simulink model "X_SimulinkModell_GUI"  (R2018b)
settings: Solver=VariableStepAuto  StartTime=0.0  StopTime=0.2  FixedStep=0.0001  RelTol=1e-3  EnableMultiTasking=on
values from neighbouring files (symbols this model uses):
  F_Normal = (m_MagPol+m_Lauferstange)*9.81    [Simulink_Rand.m]
  final_para = [-8 12 18 40 10 1 5.5 39.5 20 4 7.5 1.195 ... (5610 elements, 30x187)]    [simulink_kennfelder_altermagnet.mat]    (also in simulink_kennfelder_altermagnet_ges.mat; simulink_kennfelder_neuermagnet.mat)
  I_max = [-20 -16 -12 -8 -4 0 4 8 12 16 20]    [simulink_kennfelder_altermagnet_ges.mat]
  Kraftbedarf =     [Kraftbedarf.mat]
  Kraftbedarf_gespiegelt =     [Kraftbedarf_gespiegelt.mat]
  KraftWegStrom = KraftWegStrom'    [Simulink_Rand.m]    (also in simulink_kennfelder_altermagnet.mat = [-12.365 -12.724 -13.215 -13.344 -14.014 -14.494 -14.248 -14; simulink_kennfelder_altermagnet_ges.mat = [-12.365 -12.724 -13.215 -13.344 -14.014 -14.494 -14.248 -14; simulink_kennfelder_neuermagnet.mat = [-13.233 -13.572 -14.313 -14.247 -14.812 -15.568 -15.262 -15)
  m_Ges = m_MagPol+m_Lauferstange+m_Kupplung+m_Schaltgabel_Muffe    [Simulink_Rand.m]
  mu_haft = 1.66    [Simulink_Rand.m]
  mu_reib = 1.19    [Simulink_Rand.m]
  pos = [-8 -7 -6 -5 -4 -3 -2 -1 0 1 2 3 ... (17 elements, 1x17)]    [simulink_kennfelder_altermagnet_ges.mat]
  R_Spule = (final_para(2)+2*final_para(3)+2*final_para(6)+final_para(7))*2*pi*final_para(13)*10^(-3)*final_para(18)    [Simulink_Rand.m]
undefined symbols (not defined in the file or in its folder): Flux
libraries: simulink x4
settings Model: Creator=adp_schaltaktorik  LastModifiedBy=ohahn
settings SolverCC: ZeroCrossAlgorithm=Adaptive
settings DataIOCC: LimitDataPoints=on  SaveFormat=Array  SaveTime=off
settings OptimizationCC: LifeSpan=inf
settings DebuggingCC: IgnoredZcDiagnostic=none  SolverPrmCheckMsg=warning  MultiTaskDSMMsg=warning  MultiTaskCondExecSysMsg=none  SFUnexpectedBacktrackingDiag=warning  SFNoUnconditionalDefaultTransitionDiag=warning  SFExecutionAtInitializationDiag=none
settings HardwareCC: ProdBitPerPointer=32  ProdBitPerSizeT=32  ProdBitPerPtrDiffT=32  ProdLargestAtomicFloat=None  ProdIntDivRoundTo=Undefined  ProdEndianess=Unspecified  ProdWordSize=32  ProdHWDeviceType=32-bit Generic
settings ModelReferenceCC: PropagateSignalLabelsOutOfModel=off
settings SFSimCC: SimUseLocalCustomCode=off
settings RTWCC: RTWUseLocalCustomCode=off
settings CodeAppCC: StateflowObjectComments=on
settings GRTTargetCC: TargetLangStandard=C89/C90 (ANSI)  GeneratePreprocessorConditionals=Disable all
settings ConfigComp: CovMetricSettings=dw  CovHtmlReporting=on  CovSaveCumulativeToWorkspaceVar=on  CovSaveSingleToWorkspaceVar=on  CovExternalEMLEnable=off
settings SimscapeCC: SimscapeNormalizeSystem=off

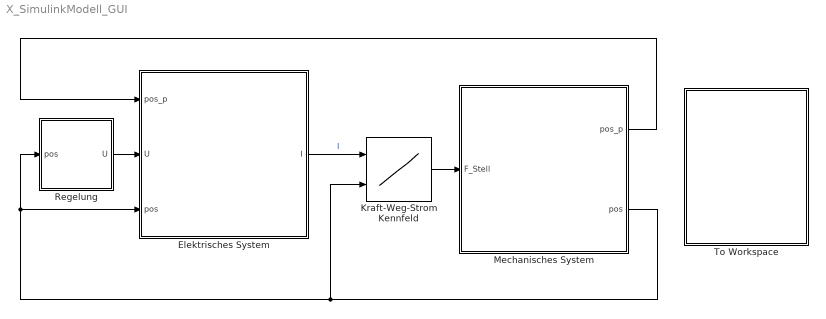
== system X_SimulinkModell_GUI ==
  Elektrisches System : Subsystem
  Kraft-Weg-Strom Kennfeld : Lookup_n-D  BreakpointsForDimension1=I_max  BreakpointsForDimension2=pos  Table=KraftWegStrom*10  InternalRulePriority=Speed  RndMeth=Simplest  InputSameDT=on
  Mechanisches System : Subsystem
  Regelung : Subsystem
  To Workspace : Subsystem
  wires:
  Mechanisches System/2(pos) -> Regelung/1("pos "), Elektrisches System/3(pos), Kraft-Weg-Strom Kennfeld/2
  Regelung/1(U) -> Elektrisches System/2(U)
  Elektrisches System/1(I) -> Kraft-Weg-Strom Kennfeld/1  "I"
  Kraft-Weg-Strom Kennfeld/1 -> Mechanisches System/1("F_Stell ")
  Mechanisches System/1("pos_p ") -> Elektrisches System/1(pos_p)

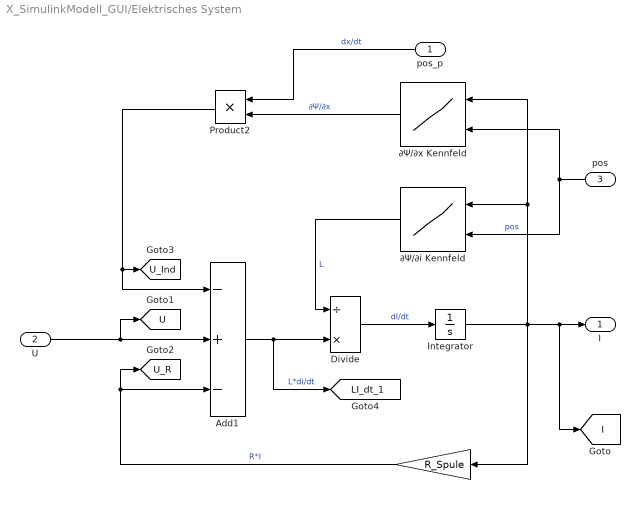
== system X_SimulinkModell_GUI/Elektrisches System ==
  pos_p : Inport
  U : Inport  Port=2
  pos : Inport  Port=3
  " " : Gain  Gain=R_Spule
  Add1 : Sum  Inputs=-+-
  Divide : Product  Inputs=/*
  Integrator : Integrator
  Product2 : Product
  "∂Ψ/∂i Kennfeld " : Lookup_n-D  BreakpointsForDimension1=Flux.i_zwischen  BreakpointsForDimension2=Flux.x  Table=Flux.phi_p_i*10  InternalRulePriority=Speed  RndMeth=Simplest  InputSameDT=on
  ∂Ψ/∂x Kennfeld : Lookup_n-D  BreakpointsForDimension1=Flux.i  BreakpointsForDimension2=Flux.x_zwischen  Table=Flux.phi_p_x*10  InternalRulePriority=Speed  RndMeth=Simplest  InputSameDT=on
  I : Outport
  tag scope: I=global, LI_dt_1=global, U=global, U_Ind=global, U_R=global
  wires:
  " "/1 -> Add1/3, [U_R]  "R*I"
  Add1/1 -> Divide/2, [LI_dt_1]  "L*di/dt"
  Divide/1 -> Integrator/1  "dI/dt"
  U/1 -> [U], Add1/2
  ∂Ψ/∂x Kennfeld/1 -> Product2/2  "∂Ψ/∂x"
  pos_p/1 -> Product2/1  "dx/dt"
  pos/1 -> "∂Ψ/∂i Kennfeld "/2, ∂Ψ/∂x Kennfeld/2  "pos"
  Product2/1 -> Add1/1, [U_Ind]
  Integrator/1 -> "∂Ψ/∂i Kennfeld "/1, ∂Ψ/∂x Kennfeld/1, [I], I/1, " "/1
  "∂Ψ/∂i Kennfeld "/1 -> Divide/1  "L"

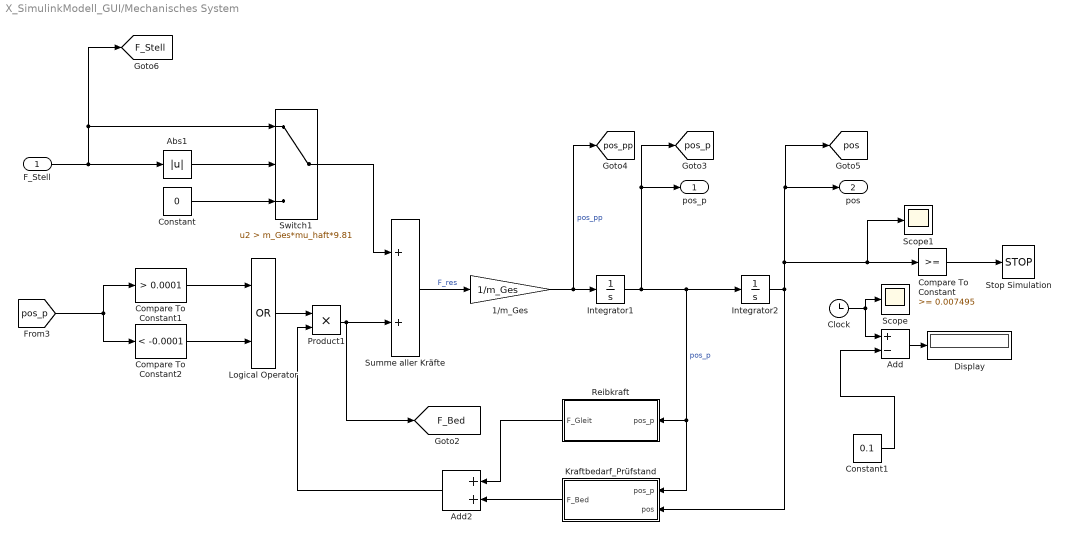
== system X_SimulinkModell_GUI/Mechanisches System ==
  "F_Stell " : Inport
  1/m_Ges : Gain  Gain=1/m_Ges
  Abs1 : Abs
  Add : Sum  Inputs=+-
  Add2 : Sum
  Clock : Clock
  Compare To Constant : simulink/Logic and Bit Operations/Compare To Constant  relop=>=  const=0.007495  OutDataTypeStr=boolean
  Compare To Constant1 : simulink/Logic and Bit Operations/Compare To Constant  relop=>  const=0.0001  OutDataTypeStr=boolean
  Compare To Constant2 : simulink/Logic and Bit Operations/Compare To Constant  relop=<  const=-0.0001  OutDataTypeStr=boolean
  Constant : Constant  Value=0
  Constant1 : Constant  Value=0.1
  Display : Display
  Integrator1 : Integrator
  Integrator2 : Integrator
  Kraftbedarf_Prüfstand : Subsystem
  Logical Operator : Logic  Operator=OR  AllPortsSameDT=off  OutDataTypeStr=boolean
  Product1 : Product
  Reibkraft : Subsystem
  Scope : Scope
  Scope1 : Scope
  Stop Simulation : Stop
  Summe aller Kräfte : Sum
  Switch1 : Switch  Criteria=u2 > Threshold  Threshold=m_Ges*mu_haft*9.81
  "pos_p " : Outport
  pos : Outport  Port=2
  tag scope: F_Bed=global, F_Stell=global, pos=global, pos_p=global, pos_pp=global
  wires:
  Integrator1/1 -> Integrator2/1, Reibkraft/1(pos_p), Kraftbedarf_Prüfstand/1(pos_p), "pos_p "/1, [pos_p]  "pos_p"
  1/m_Ges/1 -> [pos_pp], Integrator1/1  "pos_pp"
  Summe aller Kräfte/1 -> 1/m_Ges/1  "F_res"
  "F_Stell "/1 -> [F_Stell], Switch1/1, Abs1/1
  Integrator2/1 -> pos/1, [pos], Scope1/1, Compare To Constant/1, Kraftbedarf_Prüfstand/2(pos)
  Add2/1 -> Product1/2
  Abs1/1 -> Switch1/2
  Constant/1 -> Switch1/3
  Switch1/1 -> Summe aller Kräfte/1
  [pos_p] -> Compare To Constant1/1, Compare To Constant2/1
  Compare To Constant1/1 -> Logical Operator/1
  Logical Operator/1 -> Product1/1
  Reibkraft/1(F_Gleit) -> Add2/1
  Kraftbedarf_Prüfstand/1(F_Bed) -> Add2/2
  Compare To Constant2/1 -> Logical Operator/2
  Product1/1 -> [F_Bed], Summe aller Kräfte/2
  Compare To Constant/1 -> Stop Simulation/1
  Add/1 -> Display/1
  Constant1/1 -> Add/2
  Clock/1 -> Scope/1, Add/1

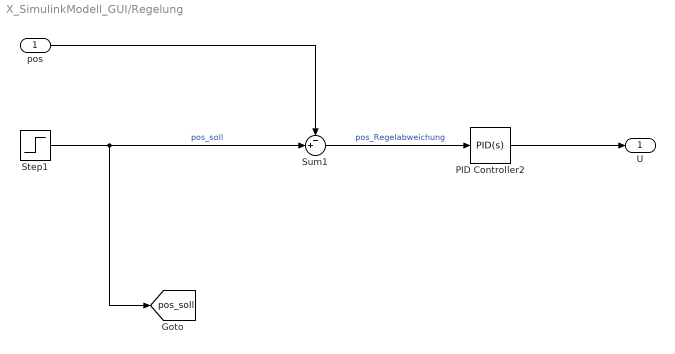
== system X_SimulinkModell_GUI/Regelung ==
  "pos " : Inport
  PID Controller2 : simulink/Continuous/PID Controller  Controller=PID  Form=Parallel  TimeDomain=Continuous-time  SampleTime=-1  IntegratorMethod=Forward Euler  FilterMethod=Forward Euler  ControllerParametersSource=internal  P=1480  I=9200  D=0  UseFilter=on  N=0  TunerSelectOption=Transfer Function Based (PID Tuner App)  InitialConditionSource=internal  InitialConditionForIntegrator=0  InitialConditionForFilter=0  DifferentiatorICPrevScaledInput=0  ExternalReset=none  TrackingMode=off  Kt=1  LimitOutput=on  UpperSaturationLimit=12  LowerSaturationLimit=-12  LinearizeAsGain=on  AntiWindupMode=none  Kb=1  POutMin=[]  POutMax=[]  IOutMin=[]  IOutMax=[]  DOutMin=[]  DOutMax=[]  NOutMin=[]  NOutMax=[]  SumOutMin=[]  SumOutMax=[]  SaturationOutMin=[]  SaturationOutMax=[]  PParamMin=[]  PParamMax=[]  IParamMin=[]  IParamMax=[]  DParamMin=[]  DParamMax=[]  NParamMin=[]  NParamMax=[]  KbParamMin=[]  KbParamMax=[]  KtParamMin=[]  KtParamMax=[]  KbOutMin=[]  KbOutMax=[]  KtOutMin=[]  KtOutMax=[]  IntegratorOutMin=[]  IntegratorOutMax=[]  FilterOutMin=[]  FilterOutMax=[]  SumI1OutMin=[]  SumI1OutMax=[]  SumI2OutMin=[]  SumI2OutMax=[]  SumI3OutMin=[]  SumI3OutMax=[]  SumI4OutMin=[]  SumI4OutMax=[]  SumDOutMin=[]  SumDOutMax=[]  DifferentiatorOutMin=[]  DifferentiatorOutMax=[]  FilterDiffOutCoefMin=[]  FilterDiffOutCoefMax=[]  ReciprocalOutMin=[]  ReciprocalOutMax=[]  SumDenOutMin=[]  SumDenOutMax=[]  SumNumOutMin=[]  SumNumOutMax=[]  DivideOutMin=[]  DivideOutMax=[]  IntegratorContinuousStateAttributes=''  IntegratorStateMustResolveToSignalObject=off  IntegratorRTWStateStorageClass=Auto  FilterContinuousStateAttributes=''  FilterStateMustResolveToSignalObject=off  FilterRTWStateStorageClass=Auto  ParallelPVariant=InternalParameters  IdealPVariant=Disabled  IVariant=InternalParameters  DVariant=InternalParameters  IntegratorVariant=Continuous  SatVariant=Enabled  AWVariant=Passthrough  PCopyVariant=Disabled  TRVariant=Disabled  FdbkBlocksVariant=Forward  IdealPFdbkVariant=Disabled  SatFdbkVariant=Disabled  DerivativeFilterVariant=ContFilter  NVariant=InternalParameters  NCopyVariant=Disabled  FilterICVariant=InternalICsFilter  IntegratorICVariant=InternalICs  ExternalResetVariant=Disabled  TRSumVariant=Passthrough  SumFdbkVariant=Disabled  SumVariant=Sum_PID
  Step1 : Step  Time=0.1  After=final_para(19)/2*0.001  SampleTime=0
  Sum1 : Sum  Inputs=-+|
  U : Outport
  tag scope: pos_soll=global
  wires:
  Step1/1 -> Sum1/2, [pos_soll]  "pos_soll"
  Sum1/1 -> PID Controller2/1  "pos_Regelabweichung"
  "pos "/1 -> Sum1/1
  PID Controller2/1 -> U/1

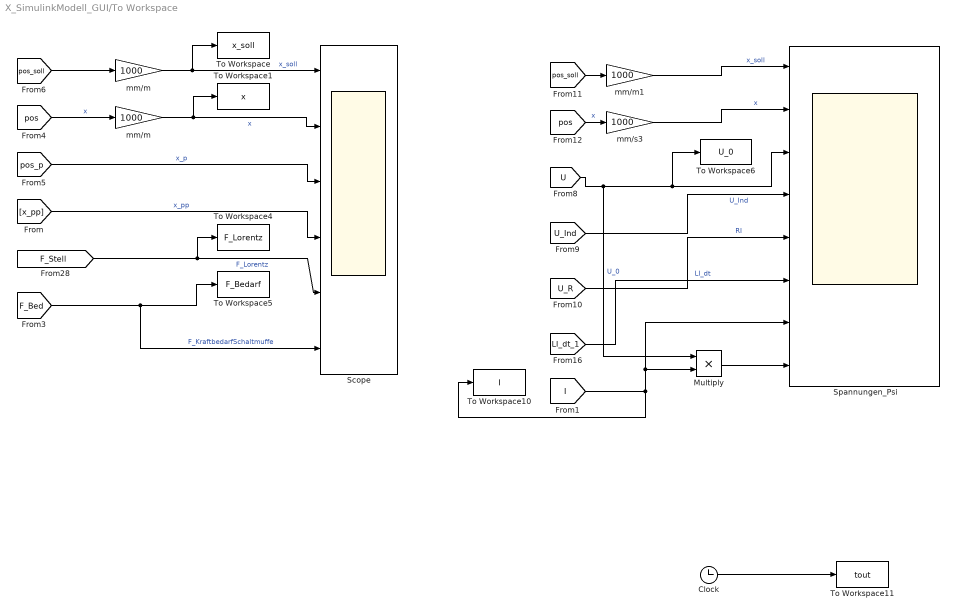
== system X_SimulinkModell_GUI/To Workspace ==
  Clock : Clock
  Multiply : Product
  Scope : Scope  NumInputPorts=6
  Spannungen_Psi : Scope  NumInputPorts=8
  To Workspace : ToWorkspace  VariableName=x_soll  SampleTime=-1
  To Workspace1 : ToWorkspace  VariableName=x  SampleTime=-1
  To Workspace10 : ToWorkspace  VariableName=I  SampleTime=-1
  To Workspace11 : ToWorkspace  VariableName=tout  SampleTime=-1
  To Workspace4 : ToWorkspace  VariableName=F_Lorentz  SampleTime=-1
  To Workspace5 : ToWorkspace  VariableName=F_Bedarf  SampleTime=-1
  To Workspace6 : ToWorkspace  VariableName=U_0  SampleTime=-1
  mm/m : Gain  Gain=1000
  "mm/m " : Gain  Gain=1000
  mm/m1 : Gain  Gain=1000
  mm/s3 : Gain  Gain=1000
  wires:
  [pos_soll] -> mm/m1/1
  [x_pp] -> Scope/4  "x_pp"
  Clock/1 -> To Workspace11/1
  [U_R] -> Spannungen_Psi/5  "RI"
  "mm/m "/1 -> Scope/2, To Workspace1/1  "x"
  [pos_p] -> Scope/3  "x_p"
  [LI_dt_1] -> Spannungen_Psi/6  "LI_dt"
  [I] -> To Workspace10/1, Multiply/2, Spannungen_Psi/7
  [F_Bed] -> To Workspace5/1, Scope/6  "F_KraftbedarfSchaltmuffe"
  [U_Ind] -> Spannungen_Psi/4  "U_Ind"
  [pos_soll] -> mm/m/1
  mm/m/1 -> Scope/1, To Workspace/1  "x_soll"
  [pos] -> mm/s3/1  "x"
  mm/m1/1 -> Spannungen_Psi/1  "x_soll"
  [U] -> Multiply/1, To Workspace6/1, Spannungen_Psi/3  "U_0"
  mm/s3/1 -> Spannungen_Psi/2  "x"
  [F_Stell] -> Scope/5, To Workspace4/1  "F_Lorentz"
  [pos] -> "mm/m "/1  "x"
  Multiply/1 -> Spannungen_Psi/8

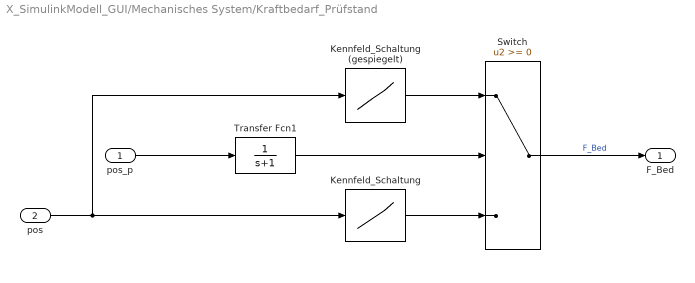
== system X_SimulinkModell_GUI/Mechanisches System/Kraftbedarf_Prüfstand ==
  pos_p : Inport
  pos : Inport  Port=2
  Kennfeld_Schaltung : Lookup_n-D  NumberOfTableDimensions=1  BreakpointsForDimension1=Kraftbedarf_gespiegelt.x*0.001  Table=-Kraftbedarf_gespiegelt.F  ExtrapMethod=Clip  UseLastTableValue=on  InternalRulePriority=Speed  RndMeth=Simplest  InputSameDT=on
  Kennfeld_Schaltung (gespiegelt) : Lookup_n-D  NumberOfTableDimensions=1  BreakpointsForDimension1=Kraftbedarf.x*0.001  Table=Kraftbedarf.F  ExtrapMethod=Clip  UseLastTableValue=on  InternalRulePriority=Speed  RndMeth=Simplest  InputSameDT=on
  Switch : Switch
  Transfer Fcn1 : TransferFcn  Denominator=[1 1]
  F_Bed : Outport
  wires:
  Kennfeld_Schaltung/1 -> Switch/3
  Kennfeld_Schaltung (gespiegelt)/1 -> Switch/1
  pos_p/1 -> Transfer Fcn1/1
  Transfer Fcn1/1 -> Switch/2
  pos/1 -> Kennfeld_Schaltung (gespiegelt)/1, Kennfeld_Schaltung/1
  Switch/1 -> F_Bed/1  "F_Bed"

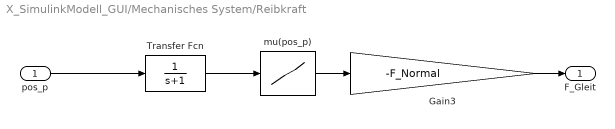
== system X_SimulinkModell_GUI/Mechanisches System/Reibkraft ==
  pos_p : Inport
  Gain3 : Gain  Gain=-F_Normal
  Transfer Fcn : TransferFcn  Denominator=[1 1]
  mu(pos_p) : Lookup_n-D  NumberOfTableDimensions=1  BreakpointsForDimension1=[-1 -0.075 -0.00001 0 0.00001 0.075 1]  Table=[-mu_reib; -mu_reib; -mu_haft; 0; mu_haft; mu_reib; mu_reib]  InterpMethod=Linear Lagrange  ExtrapMethod=Clip  UseLastTableValue=on  InternalRulePriority=Speed  RndMeth=Simplest  InputSameDT=on
  F_Gleit : Outport
  wires:
  Transfer Fcn/1 -> mu(pos_p)/1
  mu(pos_p)/1 -> Gain3/1
  pos_p/1 -> Transfer Fcn/1
  Gain3/1 -> F_Gleit/1
